simulink model "xcoilControlDesign"  (R2021a)
settings: Solver=VariableStepAuto  StartTime=0.0  StopTime=5000  FixedStep=1  RelTol=1e-3
PreLoadFcn:
  | xcoilParameters.m
undefined symbols (not defined in the file or in its folder): alpha1, am1, am2, ap1, ap2, beta1, beta2, bm, bp, k, km, kp
settings Model: Creator=b_ant  LastModifiedBy=b_ant

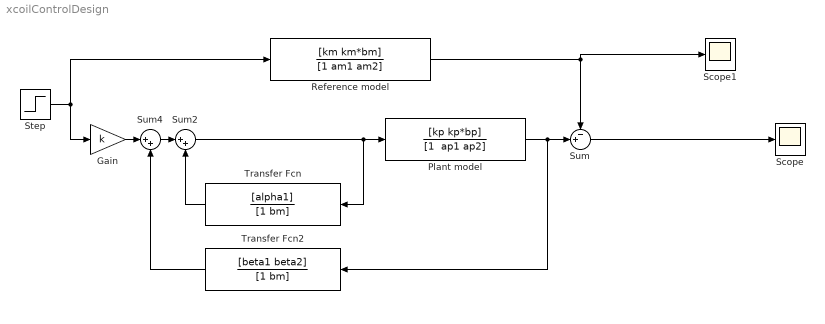
== system xcoilControlDesign ==
  Gain : Gain  Gain=k
  Plant model : TransferFcn  Numerator=[kp kp*bp]  Denominator="[1  ap1 ap2]"
  Reference model : TransferFcn  Numerator=[km km*bm]  Denominator=[1 am1 am2]
  Scope : Scope
  Scope1 : Scope
  Step : Step  SampleTime=0
  Sum : Sum  Inputs=-+|
  Sum2 : Sum  Inputs=|++
  Sum4 : Sum  Inputs=|++
  Transfer Fcn : TransferFcn  Numerator=[alpha1]  Denominator=[1 bm]
  Transfer Fcn2 : TransferFcn  Numerator=[beta1 beta2]  Denominator=[1 bm]
  wires:
  Plant model/1 -> Sum/2, Transfer Fcn2/1
  Gain/1 -> Sum4/1
  Transfer Fcn/1 -> Sum2/2
  Sum4/1 -> Sum2/1
  Sum2/1 -> Plant model/1, Transfer Fcn/1
  Transfer Fcn2/1 -> Sum4/2
  Sum/1 -> Scope/1
  Step/1 -> Reference model/1, Gain/1
  Reference model/1 -> Sum/1, Scope1/1
